simulink model "exnove"  (R2022a)
settings: Solver=VariableStepAuto  StartTime=0.0  StopTime=10.0  RelTol=1e-3
libraries: simulink x1
settings Model: Creator=a2150336  LastModifiedBy=a2150336

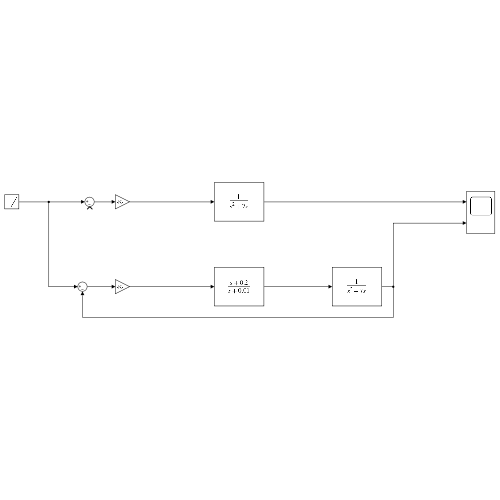
[thumbnail: Simulink's stored preview of the top-level diagram]
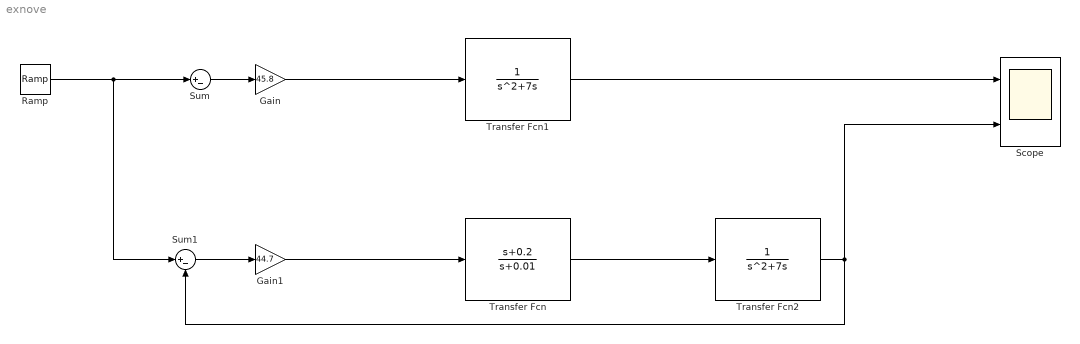
== system exnove ==
  Gain : Gain  Gain=45.8
  Gain1 : Gain  Gain=44.7
  Ramp : simulink/Sources/Ramp  slope=1  start=0  InitialOutput=0
  Scope : Scope  NumInputPorts=2
  Sum : Sum  Inputs=|+-
  Sum1 : Sum  Inputs=|+-
  Transfer Fcn : TransferFcn  Numerator=[1 0.2]  Denominator=[1 0.01]
  Transfer Fcn1 : TransferFcn  Denominator=[1 7 0]
  Transfer Fcn2 : TransferFcn  Denominator=[1 7 0]
  wires:
  Transfer Fcn/1 -> Transfer Fcn2/1
  Gain/1 -> Transfer Fcn1/1
  Gain1/1 -> Transfer Fcn/1
  Sum/1 -> Gain/1
  Ramp/1 -> Sum1/1, Sum/1
  Sum1/1 -> Gain1/1
  Transfer Fcn1/1 -> Scope/1
  Transfer Fcn2/1 -> Scope/2, Sum1/2
